simulink model "non_lin"  (R2015a)
settings: Solver=ode3  StartTime=0.0  StopTime=20  FixedStep=0.001  RelTol=1e-4
InitFcn:
  | params;
  | init_non_lin;
StopFcn:
  | visualisation_sim
values from neighbouring files (symbols this model uses):
  A1 = i_w+m_w*(R^2)+m_r*(R^2)    [init_non_lin.m]
  A2 = i_r +m_r*L^2    [init_non_lin.m]
  B1 = m_r*R*L    [init_non_lin.m]
  B2 = m_r*R*L    [init_non_lin.m]
  C1 = m_r*R*L    [init_non_lin.m]
  C2 = m_r*g*L    [init_non_lin.m]
libraries: simulink x5
settings Model: Creator=Monika  LastModifiedBy=Michał

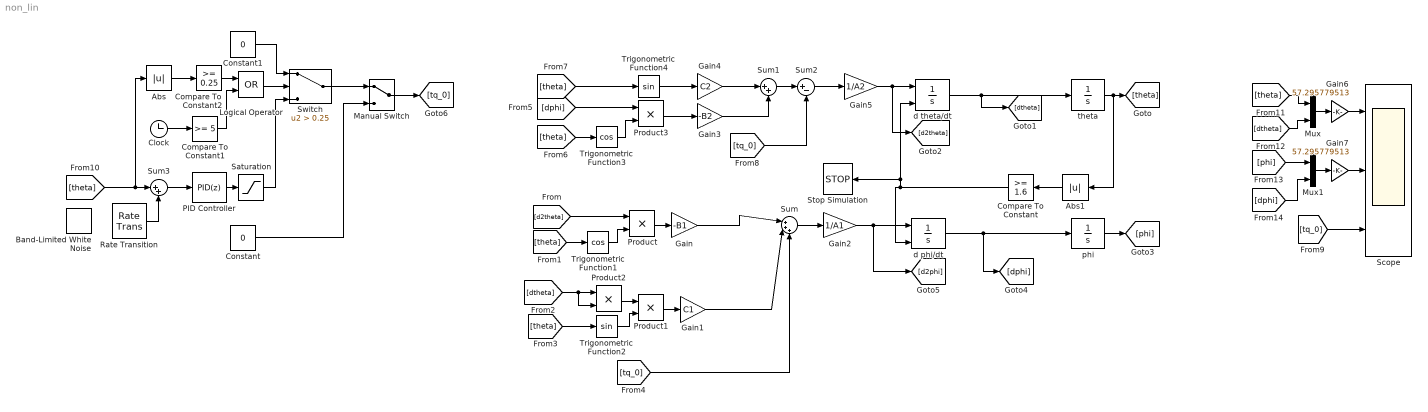
== system non_lin ==
  Abs : Abs
  Abs1 : Abs
  Band-Limited White Noise : simulink/Sources/Band-Limited White Noise  Cov=[0.0000000001]  Ts=0.001  seed=[23341]
  Clock : Clock
  Compare To Constant : simulink/Logic and Bit Operations/Compare To Constant  relop=>=  const=1.6  OutDataTypeStr=boolean
  Compare To Constant1 : simulink/Logic and Bit Operations/Compare To Constant  relop=>=  const=5  OutDataTypeStr=boolean
  Compare To Constant2 : simulink/Logic and Bit Operations/Compare To Constant  relop=>=  const=0.25  OutDataTypeStr=boolean
  Constant : Constant  Value=0
  Constant1 : Constant  Value=0
  Gain : Gain  Gain=-B1
  Gain1 : Gain  Gain=C1
  Gain2 : Gain  Gain=1/A1
  Gain3 : Gain  Gain=-B2
  Gain4 : Gain  Gain=C2
  Gain5 : Gain  Gain=1/A2
  Gain6 : Gain  Gain=57.295779513
  Gain7 : Gain  Gain=57.295779513
  Logical Operator : Logic  Operator=OR  AllPortsSameDT=off  OutDataTypeStr=boolean
  Manual Switch : ManualSwitch
  Mux : Mux  Inputs=2
  Mux1 : Mux  Inputs=2
  PID Controller : simulink/Continuous/PID Controller  Controller=PID  TimeDomain=Discrete-time  SampleTime=0.001  IntegratorMethod=Trapezoidal  FilterMethod=Forward Euler  Form=Parallel  UseFilter=off  ControllerParametersSource=internal  P=34.4904338134684  I=716.379878804257  D=0.327346067311304  N=460.807410242904  InitialConditionSource=internal  InitialConditionForIntegrator=0  InitialConditionForFilter=0  ExternalReset=none  LimitOutput=off  UpperSaturationLimit=inf  LowerSaturationLimit=-inf  LinearizeAsGain=on  AntiWindupMode=none  Kb=1  TrackingMode=off  Kt=1  PParamMin=[]  PParamMax=[]  IParamMin=[]  IParamMax=[]  DParamMin=[]  DParamMax=[]  NParamMin=[]  NParamMax=[]  KbParamMin=[]  KbParamMax=[]  KtParamMin=[]  KtParamMax=[]  POutMin=[]  POutMax=[]  IOutMin=[]  IOutMax=[]  DOutMin=[]  DOutMax=[]  NOutMin=[]  NOutMax=[]  KbOutMin=[]  KbOutMax=[]  KtOutMin=[]  KtOutMax=[]  IntegratorOutMin=[]  IntegratorOutMax=[]  FilterOutMin=[]  FilterOutMax=[]  SumOutMin=[]  SumOutMax=[]  SumI1OutMin=[]  SumI1OutMax=[]  SumI2OutMin=[]  SumI2OutMax=[]  SumI3OutMin=[]  SumI3OutMax=[]  SumDOutMin=[]  SumDOutMax=[]  SaturationOutMin=[]  SaturationOutMax=[]  IntegratorContinuousStateAttributes=''  IntegratorStateMustResolveToSignalObject=off  IntegratorRTWStateStorageClass=Auto  FilterContinuousStateAttributes=''  FilterStateMustResolveToSignalObject=off  FilterRTWStateStorageClass=Auto  DifferentiatorICPrevScaledInput=0  DifferentiatorOutMin=[]  DifferentiatorOutMax=[]
  Product{,1..3} (4 alike) : Product
  Rate Transition : RateTransition
  Saturation : Saturate  UpperLimit=175  LowerLimit=-175
  Scope : Scope  NumInputPorts=3
      settings: TimeRange=60  YMin=-2~-4~-1  YMax=8~4~1  SaveName=sim_out
  Stop Simulation : Stop
  Sum : Sum  Inputs=|+++
  Sum1 : Sum  Inputs=|++
  Sum2 : Sum  Inputs=|+-
  Sum3 : Sum  Inputs=|++
  Switch : Switch  Criteria=u2 > Threshold  Threshold=0.25
  Trigonometric Function1 : Trigonometry  Operator=cos
  Trigonometric Function2 : Trigonometry
  Trigonometric Function3 : Trigonometry  Operator=cos
  Trigonometric Function4 : Trigonometry
  d phi/dt : Integrator  ExternalReset=level  LimitOutput=on  UpperSaturationLimit=15  LowerSaturationLimit=-15
  d theta/dt : Integrator  ExternalReset=level
  phi : Integrator
  theta : Integrator  InitialCondition=0.1745329  LimitOutput=on  UpperSaturationLimit=1.6  LowerSaturationLimit=-1.6
  wires:
  theta/1 -> [theta], Abs1/1
  d theta/dt/1 -> theta/1, [dtheta]
  phi/1 -> [phi]
  d phi/dt/1 -> phi/1, [dphi]
  Product/1 -> Gain/1
  [theta] -> Trigonometric Function1/1
  Trigonometric Function1/1 -> Product/2
  [d2theta] -> Product/1
  Product1/1 -> Gain1/1
  [theta] -> Trigonometric Function2/1
  Trigonometric Function2/1 -> Product1/2
  Product2/1 -> Product1/1
  [dtheta] -> Product2/2, Product2/1
  Sum/1 -> Gain2/1
  Gain/1 -> Sum/1
  Gain1/1 -> Sum/2
  [tq_0] -> Sum/3
  Gain2/1 -> [d2phi], d phi/dt/1
  [theta] -> Trigonometric Function3/1
  [dphi] -> Product3/1
  Trigonometric Function3/1 -> Product3/2
  Product3/1 -> Gain3/1
  [theta] -> Trigonometric Function4/1
  Trigonometric Function4/1 -> Gain4/1
  Gain4/1 -> Sum1/1
  Gain3/1 -> Sum1/2
  Sum1/1 -> Sum2/1
  Sum2/1 -> Gain5/1
  [tq_0] -> Sum2/2
  Mux1/1 -> Gain7/1
  [tq_0] -> Scope/3
  Constant/1 -> Manual Switch/2
  PID Controller/1 -> Saturation/1
  Manual Switch/1 -> [tq_0]
  [theta] -> Abs/1, Sum3/1
  Sum3/1 -> PID Controller/1
  Switch/1 -> Manual Switch/1
  Saturation/1 -> Switch/3
  Abs/1 -> Compare To Constant2/1
  Constant1/1 -> Switch/1
  [theta] -> Mux/1
  [dtheta] -> Mux/2
  [phi] -> Mux1/1
  [dphi] -> Mux1/2
  Abs1/1 -> Compare To Constant/1
  Clock/1 -> Compare To Constant1/1
  Logical Operator/1 -> Switch/2
  Compare To Constant2/1 -> Logical Operator/1
  Compare To Constant1/1 -> Logical Operator/2
  Mux/1 -> Gain6/1
  Rate Transition/1 -> Sum3/2
  Gain6/1 -> Scope/1
  Gain7/1 -> Scope/2
  Gain5/1 -> [d2theta], d theta/dt/1
  Compare To Constant/1 -> Stop Simulation/1, d theta/dt/2, d phi/dt/2
